simulink model "sim_ICS2026_inv_pendulum"  (R2025b)
settings: Solver=VariableStepAuto  StartTime=0.0  StopTime=Tsim  RelTol=1e-3
values from neighbouring files (symbols this model uses):
  Ac = [0, 0, 1, 0 ... (first row only)    [main_Q21_ANN_cart_pend.m]
  Bc = [0 ... (first row only)    [main_Q21_ANN_cart_pend.m]
  g = 9.81    [main_Q21_ANN_cart_pend.m]
  mp = 0.024    [main_Q21_ANN_cart_pend.m]
  pos_ref = pi/12    (= 0.261799387799)    [main_Q21_ANN_cart_pend.m]
  ts = 1/1000    (= 0.001)    [main_Q21_ANN_cart_pend.m]
  xo = [0 0 0 0]'    [main_Q21_ANN_cart_pend.m]
undefined symbols (not defined in the file or in its folder): add_noise, bc, bp, Kv, l, Mc, pos_noise_var
settings Model: Creator=ricardoaguilera  LastModifiedBy=lskje
settings DataIOCC: ReturnWorkspaceOutputs=off
settings DebuggingCC: AlgebraicLoopMsg=none

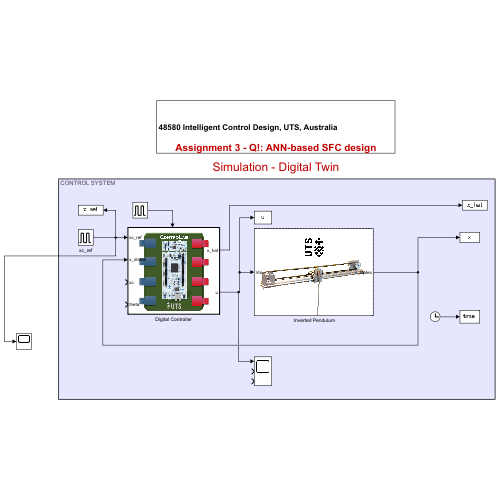
[thumbnail: Simulink's stored preview of the top-level diagram]
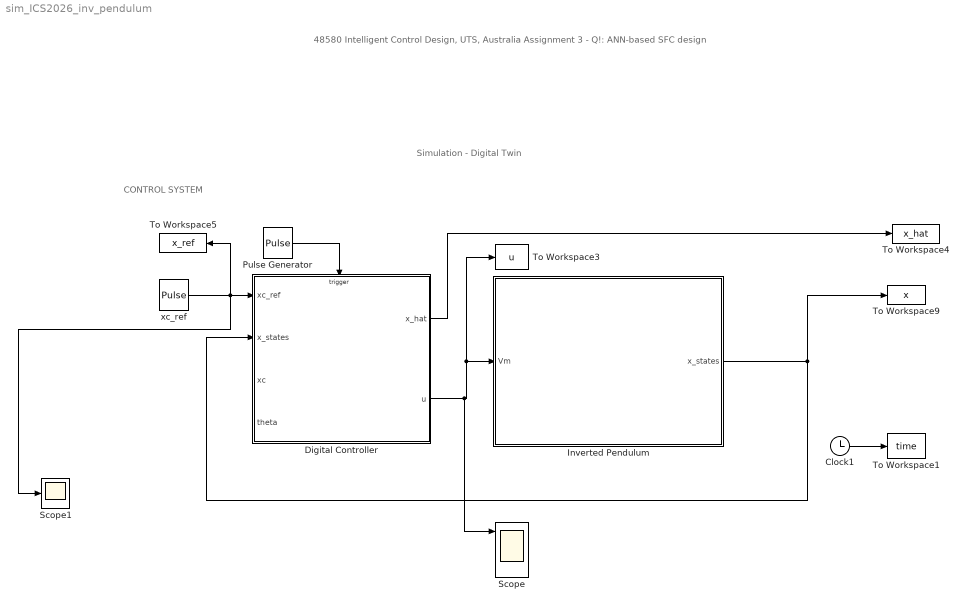
== system sim_ICS2026_inv_pendulum ==
  note: Simulation - Digital Twin
  note: 48580 Intelligent Control Design, UTS, Australia
      |
      | Assignment 3 - Q!: ANN-based SFC design
  note: CONTROL SYSTEM
  " Inverted Pendulum" : Subsystem
      mask Display: image('bitmap.png');
  Clock1 : Clock
  Digital Controller : Subsystem  TreatAsAtomicUnit=on
      mask Display: image('Controlboard.png');
  Pulse Generator : DiscretePulseGenerator  PulseType=Time based  Period=ts  PulseWidth=50
  Scope : Scope  NumInputPorts=3
      settings: ActiveDisplayYMinimum=-1  ActiveDisplayYMaximum=1
  Scope1 : Scope
      settings: ActiveDisplayYMinimum=-0.00625  ActiveDisplayYMaximum=0.05625
  To Workspace1 : ToWorkspace  VariableName=time  SampleTime=ts/100
  To Workspace3 : ToWorkspace  VariableName=u  SampleTime=ts/100
  To Workspace4 : ToWorkspace  VariableName=x_hat  SampleTime=ts/100
  To Workspace5 : ToWorkspace  VariableName=x_ref  SampleTime=ts/100
  To Workspace9 : ToWorkspace  VariableName=x  SampleTime=ts/100
  xc_ref : DiscretePulseGenerator  PulseType=Time based  Amplitude=pos_ref  Period=10  PulseWidth=50
  wires:
  Digital Controller/2(u) -> Scope/1, To Workspace3/1, " Inverted Pendulum"/1(Vm)
  Pulse Generator/1 -> Digital Controller/Trigger
  Digital Controller/1(x_hat) -> To Workspace4/1
  xc_ref/1 -> Scope1/1, To Workspace5/1, Digital Controller/1(xc_ref)
  " Inverted Pendulum"/1(x_states) -> To Workspace9/1, Digital Controller/2(x_states)
  Clock1/1 -> To Workspace1/1

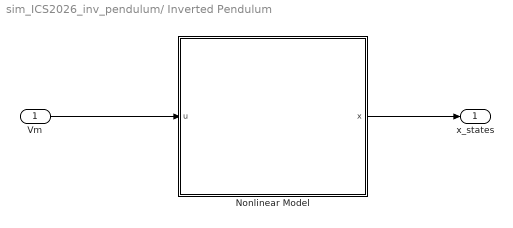
== system sim_ICS2026_inv_pendulum/ Inverted Pendulum ==
  Vm : Inport
  Nonlinear Model : Subsystem
  x_states : Outport
  wires:
  Vm/1 -> Nonlinear Model/1(u)
  Nonlinear Model/1(x) -> x_states/1

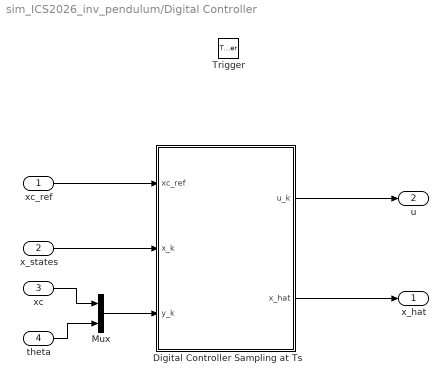
== system sim_ICS2026_inv_pendulum/Digital Controller ==
  xc_ref : Inport
  x_states : Inport  Port=2
  xc : Inport  Port=3
  theta : Inport  Port=4
  Trigger : TriggerPort  VariantControl=(inherit)  InitialTriggerSignalState=zero
  Digital Controller Sampling at Ts : MATLAB Function  TreatAsAtomicUnit=on
  Mux : Mux  Inputs=2
  x_hat : Outport
  u : Outport  Port=2
  wires:
  xc_ref/1 -> Digital Controller Sampling at Ts/1(xc_ref)
  x_states/1 -> Digital Controller Sampling at Ts/2(x_k)
  Digital Controller Sampling at Ts/1(u_k) -> u/1
  xc/1 -> Mux/1
  theta/1 -> Mux/2
  Mux/1 -> Digital Controller Sampling at Ts/3(y_k)
  Digital Controller Sampling at Ts/2(x_hat) -> x_hat/1

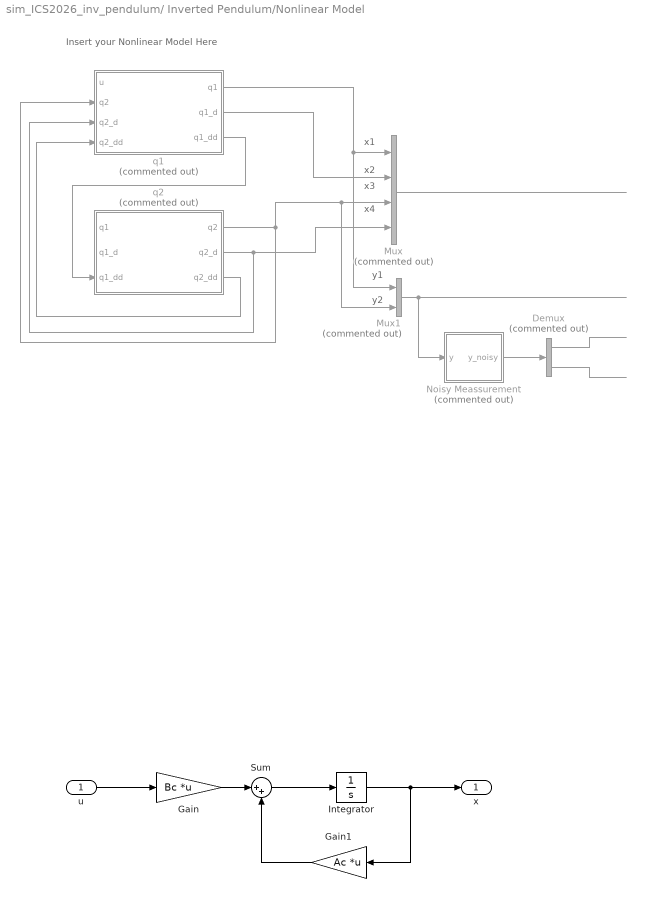
== system sim_ICS2026_inv_pendulum/ Inverted Pendulum/Nonlinear Model ==
  note: x1
  note: Insert your Nonlinear Model Here
  note: x2
  note: x3
  note: x4
  note: y1
  note: y2
  u : Inport
  Demux : Demux  Commented=on  Outputs=2
  Gain : Gain  Gain=Bc  Multiplication=Matrix(K*u)
  Gain1 : Gain  Gain=Ac  Multiplication=Matrix(K*u)
  Integrator : Integrator
  Mux : Mux  Commented=on
  Mux1 : Mux  Commented=on  Inputs=2
  Noisy Meassurement : Subsystem  Commented=on
  Sum : Sum  Inputs=|++
  q1 : Subsystem  Commented=on
  q2 : Subsystem  Commented=on
  x : Outport  VectorParamsAs1DForOutWhenUnconnected=off
  wires:
  q2/3(q2_dd) -> q1/4(q2_dd)
  q2/2(q2_d) -> q1/3(q2_d), Mux/4
  q2/1(q2) -> q1/2(q2), Mux1/2, Mux/3
  q1/2(q1_d) -> Mux/2
  q1/1(q1) -> Mux1/1, Mux/1
  Mux/1 -> ?
  Mux1/1 -> Noisy Meassurement/1(y)
  ? -> q1/1(u)
  q1/3(q1_dd) -> q2/3(q1_dd)
  Noisy Meassurement/1(y_noisy) -> Demux/1
  Demux/1 -> ?
  Demux/2 -> ?
  u/1 -> Gain/1
  Gain/1 -> Sum/1
  Sum/1 -> Integrator/1
  Integrator/1 -> Gain1/1, x/1
  Gain1/1 -> Sum/2

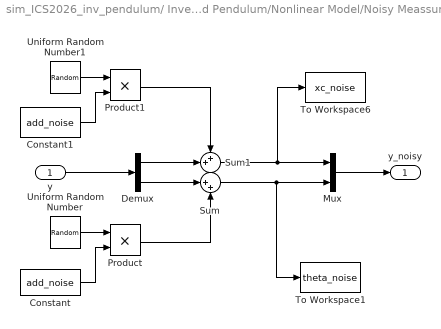
== system sim_ICS2026_inv_pendulum/ Inverted Pendulum/Nonlinear Model/Noisy Meassurement ==
  y : Inport
  Constant : Constant  Value=add_noise
  Constant1 : Constant  Value=add_noise
  Demux : Demux  Outputs=2
  Mux : Mux  Inputs=2
  Product : Product
  Product1 : Product
  Sum : Sum  Inputs=|++
  Sum1 : Sum  Inputs=++|
  To Workspace1 : ToWorkspace  VariableName=theta_noise  SampleTime=ts/100
  To Workspace6 : ToWorkspace  VariableName=xc_noise  SampleTime=ts/100
  Uniform Random Number : UniformRandomNumber  Minimum=-(0.1*pi/180)*1.8  Maximum=(0.1*pi/180)*1.8  Seed=round(rand*10)  SampleTime=ts/10
  Uniform Random Number1 : UniformRandomNumber  Minimum=-sqrt(pos_noise_var)*1.8  Maximum=sqrt(pos_noise_var)*1.8  Seed=round(rand*10)  SampleTime=ts/10
  y_noisy : Outport  VectorParamsAs1DForOutWhenUnconnected=off
  wires:
  Constant1/1 -> Product1/2
  y/1 -> Demux/1
  Mux/1 -> y_noisy/1
  Demux/1 -> Sum1/2
  Product1/1 -> Sum1/1
  Demux/2 -> Sum/1
  Product/1 -> Sum/2
  Sum1/1 -> To Workspace6/1, Mux/1
  Sum/1 -> To Workspace1/1, Mux/2
  Constant/1 -> Product/2
  Uniform Random Number/1 -> Product/1
  Uniform Random Number1/1 -> Product1/1

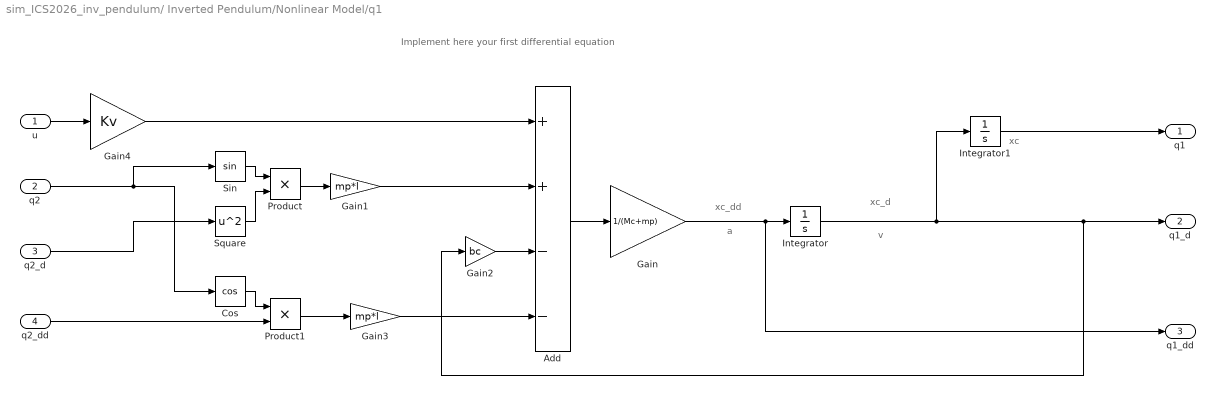
== system sim_ICS2026_inv_pendulum/ Inverted Pendulum/Nonlinear Model/q1 ==
  note: Implement here your first differential equation
  note: a
  note: xc_dd
  note: v
  note: xc_d
  note: xc
  u : Inport
  q2 : Inport  Port=2
  q2_d : Inport  Port=3
  q2_dd : Inport  Port=4
  Add : Sum  Inputs=++--
  Cos : Trigonometry  Operator=cos
  Gain : Gain  Gain=1/(Mc+mp)
  Gain1 : Gain  Gain=mp*l
  Gain2 : Gain  Gain=bc
  Gain3 : Gain  Gain=mp*l
  Gain4 : Gain  Gain=Kv
  Integrator : Integrator  InitialCondition=xo(2)
  Integrator1 : Integrator  InitialCondition=xo(1)
  Product : Product
  Product1 : Product
  Sin : Trigonometry
  Square : Math  Operator=square
  q1 : Outport  VectorParamsAs1DForOutWhenUnconnected=off
  q1_d : Outport  Port=2  VectorParamsAs1DForOutWhenUnconnected=off
  q1_dd : Outport  Port=3  VectorParamsAs1DForOutWhenUnconnected=off
  wires:
  Integrator1/1 -> q1/1
  u/1 -> Gain4/1
  Add/1 -> Gain/1
  Integrator/1 -> Gain2/1, q1_d/1, Integrator1/1
  Gain/1 -> q1_dd/1, Integrator/1
  Gain4/1 -> Add/1
  q2/1 -> Sin/1, Cos/1
  q2_d/1 -> Square/1
  Product/1 -> Gain1/1
  Square/1 -> Product/2
  Sin/1 -> Product/1
  Gain1/1 -> Add/2
  Gain2/1 -> Add/3
  Cos/1 -> Product1/1
  Gain3/1 -> Add/4
  q2_dd/1 -> Product1/2
  Product1/1 -> Gain3/1

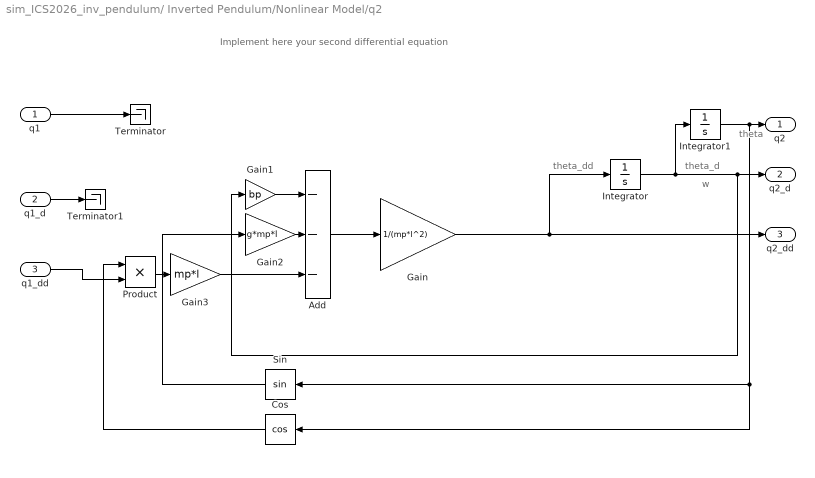
== system sim_ICS2026_inv_pendulum/ Inverted Pendulum/Nonlinear Model/q2 ==
  note: theta_dd
  note: w
  note: theta_d
  note: theta
  note: Implement here your second differential equation
  q1 : Inport
  q1_d : Inport  Port=2
  q1_dd : Inport  Port=3
  Add : Sum  Inputs=---
  Cos : Trigonometry  Operator=cos
  Gain : Gain  Gain=1/(mp*l^2)
  Gain1 : Gain  Gain=bp
  Gain2 : Gain  Gain=g*mp*l
  Gain3 : Gain  Gain=mp*l
  Integrator : Integrator  InitialCondition=xo(4)
  Integrator1 : Integrator  InitialCondition=xo(3)
  Product : Product
  Sin : Trigonometry
  Terminator : Terminator
  Terminator1 : Terminator
  q2 : Outport  VectorParamsAs1DForOutWhenUnconnected=off
  q2_d : Outport  Port=2  VectorParamsAs1DForOutWhenUnconnected=off
  q2_dd : Outport  Port=3  VectorParamsAs1DForOutWhenUnconnected=off
  wires:
  Add/1 -> Gain/1
  Integrator/1 -> Gain1/1, q2_d/1, Integrator1/1
  Gain/1 -> Integrator/1, q2_dd/1
  Integrator1/1 -> Cos/1, Sin/1, q2/1
  q1/1 -> Terminator/1
  Gain1/1 -> Add/1
  Gain2/1 -> Add/2
  Sin/1 -> Gain2/1
  q1_dd/1 -> Product/2
  Product/1 -> Gain3/1
  Gain3/1 -> Add/3
  Cos/1 -> Product/1
  q1_d/1 -> Terminator1/1

== matlab function sim_ICS2026_inv_pendulum/Digital Controller/Digital Controller Sampling at Ts ==
  data: xc_ref input; x_k input; u_k output; K_est parameter; y_k input; x_hat output
function [u_k,x_hat] = fcn(xc_ref,x_k,K_est, y_k)

%% SFC
u_k = -K_est*(x_k - xc_ref*[1 0 0 0]');

x_hat = [0 0 0 0]';
